simulink model "Test_conducting_TLS"  (R2022a)
settings: Solver=VariableStepAuto  StartTime=0.0  StopTime=1000.0  RelTol=1e-3
libraries: nesl_utility x9
settings Model: Creator=Ravi  LastModifiedBy=Ravi

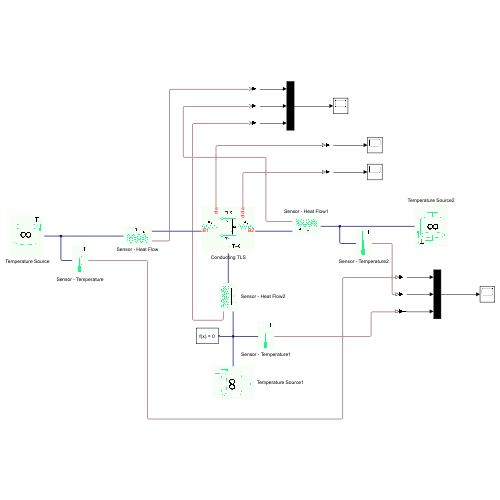
[thumbnail: Simulink's stored preview of the top-level diagram]
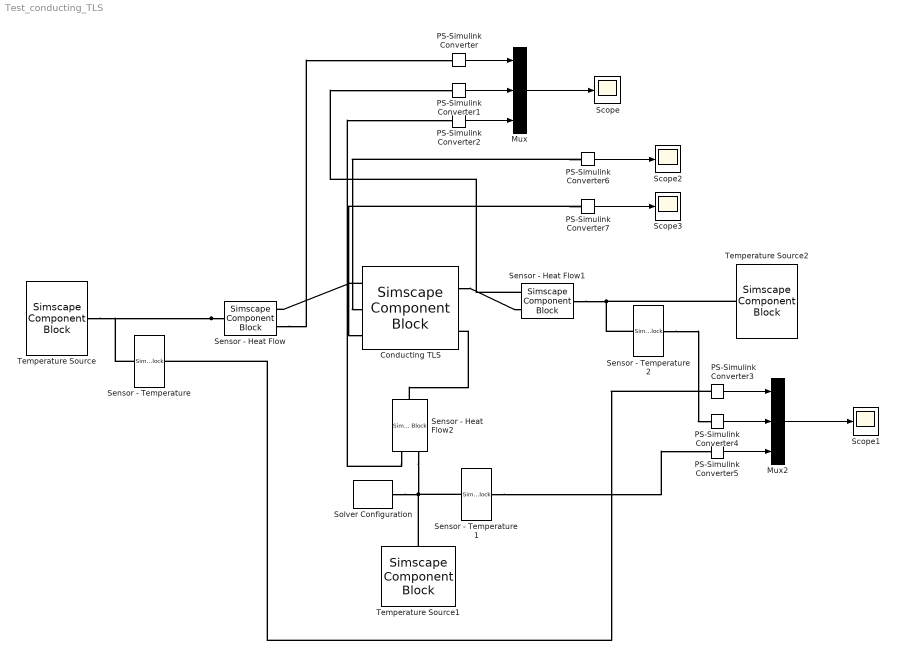
== system Test_conducting_TLS ==
  Conducting TLS : SimscapeComponentBlock  SourceFile=conducting_TLS  ComponentPath=conducting_TLS  ComponentVariants="[\"conducting_TLS\"]"  ComponentVariantNames="[\"conducting_TLS\"]"  ClassName=conducting_TLS  SchemaVersion=1  k1=0.01  k2=0.01  w=1  p11_specify=off  p11_priority=High  p11=0.5  p11_nominal_specify=off  p11_nominal_unit=1  p11_nominal_value=1  p22_specify=off  p22_priority=High  p22=0.5  p22_nominal_specify=off  p22_nominal_unit=1  p22_nominal_value=1  T1_specify=off  T1_priority=None  T1=0.2  T1_nominal_specify=off  T1_nominal_unit=1  T1_nominal_value=1  T2_specify=off  T2_priority=None  T2=0.2  T2_nominal_specify=off  T2_nominal_unit=1  T2_nominal_value=1  J1_specify=off  J1_priority=None  J1=0  J1_nominal_specify=off  J1_nominal_unit=1  J1_nominal_value=1  J2_specify=off  J2_priority=None  J2=0  J2_nominal_specify=off  J2_nominal_unit=1  J2_nominal_value=1
      settings: CopyFcn=simscape.engine.sli.internal.componentblockcallback(gcbh,'COPY')  PreCopyFcn=simscape.engine.sli.internal.componentblockcallback(gcbh,'PRECOPY')  PreDeleteFcn=simscape.engine.sli.internal.componentblockcallback(gcbh,'PREDELETE')  InternalSimscapePortConfiguration="{\"Bottom\":[{\"id\":\"gnd\",\"label\":\"\",\"type\":\"quantum_thermal\"}],\"Left\":[{\"id\":\"b1\",\"label\":\"B1\",\"type\":\"quantum_thermal\"}],\"Right\":[{\"id\":\"b2\",\"label\":\"B2\",\"type\":\"quantum_thermal\"}],\"Top\":[{\"id\":\"diag\",\"label\":\"dia\",\"type\":\"output\"},{\"id\":\"ofdiag\",\"label\":\"ofdia\",\"type\":\"output\"}]}"
      mask Type: Conducting TLS
  Mux : Mux  Inputs=3
  Mux2 : Mux  Inputs=3
  PS-Simulink Converter{,1..7} (8 alike) : nesl_utility/PS-Simulink Converter  PhysicalDomain=network_engine_domain  SubClassName=ps_output  LeftPortType=input  RightPortType=output  PseudoPeriodic=off  Frequencies=[]  VectorFormat=inherit  Unit=inherit  AffineConversion=off
      settings: SourceProductBaseCode=SS,PW,VE
  Scope{,1..3} (4 alike) : Scope
  Sensor - Heat Flow : SimscapeComponentBlock  SourceFile=sensor_heat_flow  ComponentPath=sensor_heat_flow  ComponentVariants="[\"sensor_heat_flow\"]"  ComponentVariantNames="[\"sensor_heat_flow\"]"  ClassName=sensor_heat_flow  SchemaVersion=1  J_specify=off  J_priority=None  J=0  J_nominal_specify=off  J_nominal_unit=1  J_nominal_value=1
      settings: CopyFcn=simscape.engine.sli.internal.componentblockcallback(gcbh,'COPY')  PreCopyFcn=simscape.engine.sli.internal.componentblockcallback(gcbh,'PRECOPY')  PreDeleteFcn=simscape.engine.sli.internal.componentblockcallback(gcbh,'PREDELETE')  InternalSimscapePortConfiguration="{\"Bottom\":[],\"Left\":[{\"id\":\"inp\",\"label\":\"\",\"type\":\"quantum_thermal\"}],\"Right\":[{\"id\":\"out\",\"label\":\"\",\"type\":\"quantum_thermal\"},{\"id\":\"sense\",\"label\":\"\",\"type\":\"output\"}],\"Top\":[]}"
      mask Type: Heat flow rate sensor
  Sensor - Heat Flow1 : SimscapeComponentBlock  SourceFile=sensor_heat_flow  ComponentPath=sensor_heat_flow  ComponentVariants="[\"sensor_heat_flow\"]"  ComponentVariantNames="[\"sensor_heat_flow\"]"  ClassName=sensor_heat_flow  SchemaVersion=1  J_specify=off  J_priority=None  J=0  J_nominal_specify=off  J_nominal_unit=1  J_nominal_value=1
      settings: CopyFcn=simscape.engine.sli.internal.componentblockcallback(gcbh,'COPY')  PreCopyFcn=simscape.engine.sli.internal.componentblockcallback(gcbh,'PRECOPY')  PreDeleteFcn=simscape.engine.sli.internal.componentblockcallback(gcbh,'PREDELETE')  InternalSimscapePortConfiguration="{\"Bottom\":[],\"Left\":[{\"id\":\"inp\",\"label\":\"\",\"type\":\"quantum_thermal\"}],\"Right\":[{\"id\":\"out\",\"label\":\"\",\"type\":\"quantum_thermal\"},{\"id\":\"sense\",\"label\":\"\",\"type\":\"output\"}],\"Top\":[]}"
      mask Type: Heat flow rate sensor
  Sensor - Heat Flow2 : SimscapeComponentBlock  SourceFile=sensor_heat_flow  ComponentPath=sensor_heat_flow  ComponentVariants="[\"sensor_heat_flow\"]"  ComponentVariantNames="[\"sensor_heat_flow\"]"  ClassName=sensor_heat_flow  SchemaVersion=1  J_specify=off  J_priority=None  J=0  J_nominal_specify=off  J_nominal_unit=1  J_nominal_value=1
      settings: CopyFcn=simscape.engine.sli.internal.componentblockcallback(gcbh,'COPY')  PreCopyFcn=simscape.engine.sli.internal.componentblockcallback(gcbh,'PRECOPY')  PreDeleteFcn=simscape.engine.sli.internal.componentblockcallback(gcbh,'PREDELETE')  InternalSimscapePortConfiguration="{\"Bottom\":[],\"Left\":[{\"id\":\"inp\",\"label\":\"\",\"type\":\"quantum_thermal\"}],\"Right\":[{\"id\":\"out\",\"label\":\"\",\"type\":\"quantum_thermal\"},{\"id\":\"sense\",\"label\":\"\",\"type\":\"output\"}],\"Top\":[]}"
      mask Type: Heat flow rate sensor
  Sensor - Temperature : SimscapeComponentBlock  SourceFile=sensor_temperature  ComponentPath=sensor_temperature  ComponentVariants="[\"sensor_temperature\"]"  ComponentVariantNames="[\"sensor_temperature\"]"  ClassName=sensor_temperature  SchemaVersion=1  J_specify=off  J_priority=None  J=0  J_nominal_specify=off  J_nominal_unit=1  J_nominal_value=1
      settings: CopyFcn=simscape.engine.sli.internal.componentblockcallback(gcbh,'COPY')  PreCopyFcn=simscape.engine.sli.internal.componentblockcallback(gcbh,'PRECOPY')  PreDeleteFcn=simscape.engine.sli.internal.componentblockcallback(gcbh,'PREDELETE')  InternalSimscapePortConfiguration="{\"Bottom\":[],\"Left\":[{\"id\":\"inp\",\"label\":\"\",\"type\":\"quantum_thermal\"}],\"Right\":[{\"id\":\"sense\",\"label\":\"\",\"type\":\"output\"}],\"Top\":[]}"
      mask Type: Temperature sensor
  Sensor - Temperature1 : SimscapeComponentBlock  SourceFile=sensor_temperature  ComponentPath=sensor_temperature  ComponentVariants="[\"sensor_temperature\"]"  ComponentVariantNames="[\"sensor_temperature\"]"  ClassName=sensor_temperature  SchemaVersion=1  J_specify=off  J_priority=None  J=0  J_nominal_specify=off  J_nominal_unit=1  J_nominal_value=1
      settings: CopyFcn=simscape.engine.sli.internal.componentblockcallback(gcbh,'COPY')  PreCopyFcn=simscape.engine.sli.internal.componentblockcallback(gcbh,'PRECOPY')  PreDeleteFcn=simscape.engine.sli.internal.componentblockcallback(gcbh,'PREDELETE')  InternalSimscapePortConfiguration="{\"Bottom\":[],\"Left\":[{\"id\":\"inp\",\"label\":\"\",\"type\":\"quantum_thermal\"}],\"Right\":[{\"id\":\"sense\",\"label\":\"\",\"type\":\"output\"}],\"Top\":[]}"
      mask Type: Temperature sensor
  Sensor - Temperature2 : SimscapeComponentBlock  SourceFile=sensor_temperature  ComponentPath=sensor_temperature  ComponentVariants="[\"sensor_temperature\"]"  ComponentVariantNames="[\"sensor_temperature\"]"  ClassName=sensor_temperature  SchemaVersion=1  J_specify=off  J_priority=None  J=0  J_nominal_specify=off  J_nominal_unit=1  J_nominal_value=1
      settings: CopyFcn=simscape.engine.sli.internal.componentblockcallback(gcbh,'COPY')  PreCopyFcn=simscape.engine.sli.internal.componentblockcallback(gcbh,'PRECOPY')  PreDeleteFcn=simscape.engine.sli.internal.componentblockcallback(gcbh,'PREDELETE')  InternalSimscapePortConfiguration="{\"Bottom\":[],\"Left\":[{\"id\":\"inp\",\"label\":\"\",\"type\":\"quantum_thermal\"}],\"Right\":[{\"id\":\"sense\",\"label\":\"\",\"type\":\"output\"}],\"Top\":[]}"
      mask Type: Temperature sensor
  Solver Configuration : nesl_utility/Solver Configuration  PhysicalDomain=network_engine_domain  SubClassName=solver  LeftPortType=input  RightPortType=generic  Tones=[]  Harmonics=[]  SimulateNoise=off  Profile=off  UseLocalSampling=off  EnableSwitchedLinearOptims=on  FrequencyDomain=off  UseCCode=off  RelTol=0.001  AbsTol=0.001  MinStep=1e-09  ToWorkspace=off  RevertToSquareIcSolve=off  NumHomotopyIterations=100  PhasorMode=off  PhasorModeNumHarmonics=1  IndexReductionMethod=DerivativeReplacement  DoDC=off  ResidualTolerance=1e-09  UseLocalSolver=off  LocalSolverChoice=NE_BACKWARD_EULER_ADVANCER  LocalSolverSampleTime=0.001  DoFixedCost=off  MaxNonlinIter=3  MaxModeIter=2  ComputeImpulses=off  ImpulseIterations=2  LinearAlgebra=auto  LinearAlgebraNumThread=0  EquationFormulation=NE_TIME_EF  DelaysMemoryBudget=1024  AutomaticFiltering=on  FilteringTimeConstant=0.001  PartitionStorageMethod=AS_NEEDED  PartitionMemoryBudget=1024  PartitionMethod=ROBUST
      settings: SourceProductBaseCode=SS,PW,VE
  Temperature Source : SimscapeComponentBlock  SourceFile=source_temperature  ComponentPath=source_temperature  ComponentVariants="[\"source_temperature\"]"  ComponentVariantNames="[\"source_temperature\"]"  ClassName=source_temperature  SchemaVersion=1  temp=0.2  J_specify=off  J_priority=None  J=0  J_nominal_specify=off  J_nominal_unit=1  J_nominal_value=1
      settings: CopyFcn=simscape.engine.sli.internal.componentblockcallback(gcbh,'COPY')  PreCopyFcn=simscape.engine.sli.internal.componentblockcallback(gcbh,'PRECOPY')  PreDeleteFcn=simscape.engine.sli.internal.componentblockcallback(gcbh,'PREDELETE')  InternalSimscapePortConfiguration="{\"Bottom\":[],\"Left\":[],\"Right\":[{\"id\":\"out\",\"label\":\"\",\"type\":\"quantum_thermal\"}],\"Top\":[]}"
      mask Type: Temperature source
  Temperature Source1 : SimscapeComponentBlock  SourceFile=source_temperature  ComponentPath=source_temperature  ComponentVariants="[\"source_temperature\"]"  ComponentVariantNames="[\"source_temperature\"]"  ClassName=source_temperature  SchemaVersion=1  temp=0  J_specify=off  J_priority=None  J=0  J_nominal_specify=off  J_nominal_unit=1  J_nominal_value=1
      settings: CopyFcn=simscape.engine.sli.internal.componentblockcallback(gcbh,'COPY')  PreCopyFcn=simscape.engine.sli.internal.componentblockcallback(gcbh,'PRECOPY')  PreDeleteFcn=simscape.engine.sli.internal.componentblockcallback(gcbh,'PREDELETE')  InternalSimscapePortConfiguration="{\"Bottom\":[],\"Left\":[],\"Right\":[{\"id\":\"out\",\"label\":\"\",\"type\":\"quantum_thermal\"}],\"Top\":[]}"
      mask Type: Temperature source
  Temperature Source2 : SimscapeComponentBlock  SourceFile=source_temperature  ComponentPath=source_temperature  ComponentVariants="[\"source_temperature\"]"  ComponentVariantNames="[\"source_temperature\"]"  ClassName=source_temperature  SchemaVersion=1  temp=0.02  J_specify=off  J_priority=None  J=0  J_nominal_specify=off  J_nominal_unit=1  J_nominal_value=1
      settings: CopyFcn=simscape.engine.sli.internal.componentblockcallback(gcbh,'COPY')  PreCopyFcn=simscape.engine.sli.internal.componentblockcallback(gcbh,'PRECOPY')  PreDeleteFcn=simscape.engine.sli.internal.componentblockcallback(gcbh,'PREDELETE')  InternalSimscapePortConfiguration="{\"Bottom\":[],\"Left\":[],\"Right\":[{\"id\":\"out\",\"label\":\"\",\"type\":\"quantum_thermal\"}],\"Top\":[]}"
      mask Type: Temperature source
  wires:
  PS-Simulink Converter5/1 -> Mux2/3
  PS-Simulink Converter4/1 -> Mux2/2
  PS-Simulink Converter3/1 -> Mux2/1
  PS-Simulink Converter2/1 -> Mux/3
  PS-Simulink Converter1/1 -> Mux/2
  PS-Simulink Converter/1 -> Mux/1
  Mux/1 -> Scope/1
  Mux2/1 -> Scope1/1
  PS-Simulink Converter6/1 -> Scope2/1
  PS-Simulink Converter7/1 -> Scope3/1
  connections:
  Sensor - Heat Flow/LConn1 -- Temperature Source/RConn1 -- Sensor - Temperature/LConn1
  Conducting TLS/LConn1 -- Sensor - Heat Flow/RConn1
  Sensor - Heat Flow1/LConn1 -- Temperature Source2/RConn1 -- Sensor - Temperature2/LConn1
  Conducting TLS/RConn1 -- Sensor - Heat Flow1/RConn1
  Sensor - Heat Flow2/RConn1 -- Temperature Source1/RConn1 -- Sensor - Temperature1/LConn1 -- Solver Configuration/RConn1
  PS-Simulink Converter3/LConn1 -- Sensor - Temperature/RConn1
  Sensor - Temperature2/RConn1 -- PS-Simulink Converter4/LConn1
  Sensor - Temperature1/RConn1 -- PS-Simulink Converter5/LConn1
  Sensor - Heat Flow/RConn2 -- PS-Simulink Converter/LConn1
  Sensor - Heat Flow1/RConn2 -- PS-Simulink Converter1/LConn1
  Sensor - Heat Flow2/RConn2 -- PS-Simulink Converter2/LConn1
  PS-Simulink Converter6/LConn1 -- Conducting TLS/LConn2
  PS-Simulink Converter7/LConn1 -- Conducting TLS/LConn3
  Sensor - Heat Flow2/LConn1 -- Conducting TLS/RConn2
